simulink model "TBRe19_ECU_Torque_request_TSS_ON"  (R2017b)
settings: Solver=FixedStepDiscrete  StartTime=0.0  StopTime=inf  FixedStep=0.0001  RelTol=1e-3
PostLoadFcn:
  | model_init();
libraries: simulink x17
(part 2 of 6)

== system TBRe19_ECU_Torque_request_TSS_ON/MainTask/Comms_And_Data_Acquisition_Layer/MCU_CAN ==
  note: Overall Functionality:
      | Read CAN messages related to motor control unit (MCU)
  Bus Creator1 : BusCreator  Inputs=4
  CanRx1 : S-Function  FunctionName=NsiCan_Rx_J1939_Ext  Parameters=data_can,channel,msg_name,ident,ident_type,dlc,signals,is_trigger,is_SA_Masked,is_TA_Masked,is_physical,is_canfd  SFunctionDeploymentMode=off  EnableBusSupport=off  mask(MUXlink Can Rx){data_can=1;HIGH_SPEED;500Kbps;No;C:\Users\TBRe-admin\Documents\TBReVCU\TBRe19_DBC.dbc;0;;;0;HIGH_SPEED;500Kbps;120 Ohm;C:\Users\TBRe-admin\Documents\Database\TBRe19_DBC_190517.dbc;0;;;0;HIGH_SPEED;1000Kbps;120 Ohm;D:\TOOLS\MUXLINK\R2011b\MUXlink\misc\BASE_CAN_MUXLAB4.dbc;0;;;0;HIGH_SPEED;500Kbps;120 Ohm;D:\TOOLS\MUXLINK\R2011b\MUXlink\misc\j1939_adapt.dbc;0;;;0;HIGH_SPEED;1000Kbps;No;D:\TOOLS\MUXLINK\R2011b\MUXlink\misc\BASE_CAN_MUXLAB4.dbc;0;;, channel=1, msg_name=HS3_Temperature_Feedback, ident=0x191AFF71, ident_type=XTD, dlc=8, signals=DC_Link_Voltage;1;32;-16;0.062500;0.000000;V;MotorTemperature;1;16;-16;1.000000;0.000000;C, is_trigger=0, is_physical=1, is_canfd=0, is_SA_Masked=1, is_TA_Masked=0}
      mask prompts: data_can "data can"; msg_name "msg name"; is_SA_Masked "J1939 SA filtering"; is_TA_Masked "J1939 TA filtering"
      mask help: Receive a frame from a CAN channel.
      mask init:
      | NsiCan_Rx_J1939_Ext_InitializationFcn();
      settings: OpenFcn=NsiCan_Rx_J1939_Ext_OpenFcn();
      mask Help:
      | eval('block=get_param(gcb, ''RTWdata'');')
      | web([docroot '\toolbox\MUXlink\html\blocks/' block.MUXlink_BlockType '.html'])
      mask Callback data_can: NsiCan_Rx_J1939_Ext_ApplyFcn(1);
      mask Callback channel: NsiCan_Rx_J1939_Ext_ApplyFcn(2);
      mask Callback msg_name: NsiCan_Rx_J1939_Ext_ApplyFcn(3);
      mask Callback ident: NsiCan_Rx_J1939_Ext_ApplyFcn(4);
      mask Callback ident_type: NsiCan_Rx_J1939_Ext_ApplyFcn(5);
      mask Callback dlc: NsiCan_Rx_J1939_Ext_ApplyFcn(6);
      mask Callback signals: NsiCan_Rx_J1939_Ext_ApplyFcn(7);
      mask Callback is_trigger: NsiCan_Rx_J1939_Ext_ApplyFcn(8);
      mask Callback is_physical: NsiCan_Rx_J1939_Ext_ApplyFcn(9);
      mask Callback is_canfd: NsiCan_Rx_J1939_Ext_ApplyFcn(10);
      mask Callback is_SA_Masked: NsiCan_Rx_J1939_Ext_ApplyFcn(11);
      mask Callback is_TA_Masked: NsiCan_Rx_J1939_Ext_ApplyFcn(12);
      mask Display: image(imread('nsi.bmp'));text(0.5, 0.3, 'J1939_PGN  HS3_Temperature_Feedbackchannel CAN1', 'horizontalAlignment', 'center', 'verticalAlignment', 'base');plot([0.05 0.05 0.05 0.05 0.05 0.05 0.05 0.05 0.05 0.05]); port_label('output',1, 'DC_Link_Voltage'); port_label('output',2, 'MotorTemperature'); port_label('output',3, 'Status');
  CanRx2 : S-Function  FunctionName=NsiCan_Rx_J1939_Ext  Parameters=data_can,channel,msg_name,ident,ident_type,dlc,signals,is_trigger,is_SA_Masked,is_TA_Masked,is_physical,is_canfd  SFunctionDeploymentMode=off  EnableBusSupport=off  mask(MUXlink Can Rx){data_can=1;HIGH_SPEED;500Kbps;No;C:\Users\TBRe-admin\Documents\TBReVCU\TBRe19_DBC.dbc;0;;;0;HIGH_SPEED;500Kbps;120 Ohm;C:\Users\TBRe-admin\Documents\Database\TBRe19_DBC_190517.dbc;0;;;0;HIGH_SPEED;1000Kbps;120 Ohm;D:\TOOLS\MUXLINK\R2011b\MUXlink\misc\BASE_CAN_MUXLAB4.dbc;0;;;0;HIGH_SPEED;500Kbps;120 Ohm;D:\TOOLS\MUXLINK\R2011b\MUXlink\misc\j1939_adapt.dbc;0;;;0;HIGH_SPEED;1000Kbps;No;D:\TOOLS\MUXLINK\R2011b\MUXlink\misc\BASE_CAN_MUXLAB4.dbc;0;;, channel=1, msg_name=HD4_Debug_Temperatures_B, ident=0x192BFF71, ident_type=XTD, dlc=8, signals=Debug_Temps_Heatsink;1;24;8;1.000000;0.000000;degC, is_trigger=0, is_physical=1, is_canfd=0, is_SA_Masked=1, is_TA_Masked=0}
      mask prompts: data_can "data can"; msg_name "msg name"; is_SA_Masked "J1939 SA filtering"; is_TA_Masked "J1939 TA filtering"
      mask help: Receive a frame from a CAN channel.
      mask init:
      | NsiCan_Rx_J1939_Ext_InitializationFcn();
      settings: OpenFcn=NsiCan_Rx_J1939_Ext_OpenFcn();
      mask Help:
      | eval('block=get_param(gcb, ''RTWdata'');')
      | web([docroot '\toolbox\MUXlink\html\blocks/' block.MUXlink_BlockType '.html'])
      mask Callback data_can: NsiCan_Rx_J1939_Ext_ApplyFcn(1);
      mask Callback channel: NsiCan_Rx_J1939_Ext_ApplyFcn(2);
      mask Callback msg_name: NsiCan_Rx_J1939_Ext_ApplyFcn(3);
      mask Callback ident: NsiCan_Rx_J1939_Ext_ApplyFcn(4);
      mask Callback ident_type: NsiCan_Rx_J1939_Ext_ApplyFcn(5);
      mask Callback dlc: NsiCan_Rx_J1939_Ext_ApplyFcn(6);
      mask Callback signals: NsiCan_Rx_J1939_Ext_ApplyFcn(7);
      mask Callback is_trigger: NsiCan_Rx_J1939_Ext_ApplyFcn(8);
      mask Callback is_physical: NsiCan_Rx_J1939_Ext_ApplyFcn(9);
      mask Callback is_canfd: NsiCan_Rx_J1939_Ext_ApplyFcn(10);
      mask Callback is_SA_Masked: NsiCan_Rx_J1939_Ext_ApplyFcn(11);
      mask Callback is_TA_Masked: NsiCan_Rx_J1939_Ext_ApplyFcn(12);
      mask Display: image(imread('nsi.bmp'));text(0.5, 0.3, 'J1939_PGN  HD4_Debug_Temperatures_Bchannel CAN1', 'horizontalAlignment', 'center', 'verticalAlignment', 'base');plot([0.05 0.05 0.05 0.05 0.05 0.05 0.05 0.05 0.05 0.05]); port_label('output',1, 'Debug_Temps_Heatsink'); port_label('output',2, 'Status');
  CanRx3 : S-Function  FunctionName=NsiCan_Rx_J1939_Ext  Parameters=data_can,channel,msg_name,ident,ident_type,dlc,signals,is_trigger,is_SA_Masked,is_TA_Masked,is_physical,is_canfd  SFunctionDeploymentMode=off  EnableBusSupport=off  mask(MUXlink Can Rx){data_can=1;HIGH_SPEED;500Kbps;No;C:\Users\TBRe-admin\Documents\TBReVCU\TBRe19_DBC.dbc;0;;;0;HIGH_SPEED;500Kbps;120 Ohm;C:\Users\TBRe-admin\Documents\Database\TBRe19_DBC_190517.dbc;0;;;0;HIGH_SPEED;1000Kbps;120 Ohm;D:\TOOLS\MUXLINK\R2011b\MUXlink\misc\BASE_CAN_MUXLAB4.dbc;0;;;0;HIGH_SPEED;500Kbps;120 Ohm;D:\TOOLS\MUXLINK\R2011b\MUXlink\misc\j1939_adapt.dbc;0;;;0;HIGH_SPEED;1000Kbps;No;D:\TOOLS\MUXLINK\R2011b\MUXlink\misc\BASE_CAN_MUXLAB4.dbc;0;;, channel=1, msg_name=HS1_Torque_Feedback, ident=0x1918FF71, ident_type=XTD, dlc=8, signals=Speed_Measured;1;16;-16;1.000000;0.000000;RPM;Torque_Measured;1;0;-16;0.062500;0.000000;Nm, is_trigger=0, is_physical=1, is_canfd=0, is_SA_Masked=1, is_TA_Masked=0}
      mask prompts: data_can "data can"; msg_name "msg name"; is_SA_Masked "J1939 SA filtering"; is_TA_Masked "J1939 TA filtering"
      mask help: Receive a frame from a CAN channel.
      mask init:
      | NsiCan_Rx_J1939_Ext_InitializationFcn();
      settings: OpenFcn=NsiCan_Rx_J1939_Ext_OpenFcn();
      mask Help:
      | eval('block=get_param(gcb, ''RTWdata'');')
      | web([docroot '\toolbox\MUXlink\html\blocks/' block.MUXlink_BlockType '.html'])
      mask Callback data_can: NsiCan_Rx_J1939_Ext_ApplyFcn(1);
      mask Callback channel: NsiCan_Rx_J1939_Ext_ApplyFcn(2);
      mask Callback msg_name: NsiCan_Rx_J1939_Ext_ApplyFcn(3);
      mask Callback ident: NsiCan_Rx_J1939_Ext_ApplyFcn(4);
      mask Callback ident_type: NsiCan_Rx_J1939_Ext_ApplyFcn(5);
      mask Callback dlc: NsiCan_Rx_J1939_Ext_ApplyFcn(6);
      mask Callback signals: NsiCan_Rx_J1939_Ext_ApplyFcn(7);
      mask Callback is_trigger: NsiCan_Rx_J1939_Ext_ApplyFcn(8);
      mask Callback is_physical: NsiCan_Rx_J1939_Ext_ApplyFcn(9);
      mask Callback is_canfd: NsiCan_Rx_J1939_Ext_ApplyFcn(10);
      mask Callback is_SA_Masked: NsiCan_Rx_J1939_Ext_ApplyFcn(11);
      mask Callback is_TA_Masked: NsiCan_Rx_J1939_Ext_ApplyFcn(12);
      mask Display: image(imread('nsi.bmp'));text(0.5, 0.3, 'J1939_PGN  HS1_Torque_Feedbackchannel CAN1', 'horizontalAlignment', 'center', 'verticalAlignment', 'base');plot([0.05 0.05 0.05 0.05 0.05 0.05 0.05 0.05 0.05 0.05]); port_label('output',1, 'Speed_Measured'); port_label('output',2, 'Torque_Measured'); port_label('output',3, 'Status');
  Data Type Conversion : DataTypeConversion  OutDataTypeStr=int16
  Terminator : Terminator
  Terminator1 : Terminator
  Terminator2 : Terminator
  UsbTx1 : S-Function  FunctionName=NsiUsb_Tx  Parameters=signame,resolution,offset,unite  SFunctionDeploymentMode=off  EnableBusSupport=off  mask(MUXlink Usb Tx){signame=MCU_V, resolution=1, offset=0, unite=V}
      mask prompts: signame "Signal name ?"; resolution "Resolution ?"; offset "Offset ?"; unite "Unit ?"
      mask help: Transmit a frame on the USB Channel.
      mask init:
      | NsiUsb_Tx_InitializationFcn();
      settings: OpenFcn=NsiUsb_Tx_OpenFcn();
      mask Help:
      | eval('block=get_param(gcb, ''RTWdata'');')
      | web([docroot '\toolbox\MUXlink\html\blocks/' block.MUXlink_BlockType '.html'])
      mask Callback signame: NsiUsb_Tx_ApplyFcn(1);
      mask Callback resolution: NsiUsb_Tx_ApplyFcn(2);
      mask Callback offset: NsiUsb_Tx_ApplyFcn(3);
      mask Callback unite: NsiUsb_Tx_ApplyFcn(4);
      mask Display: image(imread('nsi.bmp'));text(0.5, 0.2, 'USB Tx', 'horizontalAlignment', 'center', 'verticalAlignment', 'base');plot([0.05 0.05 0.05 0.05 0.05 0.05 0.05 0.05 0.05 0.05]);port_label('input',1, 'MCU_V');
  UsbTx2 : S-Function  FunctionName=NsiUsb_Tx  Parameters=signame,resolution,offset,unite  SFunctionDeploymentMode=off  EnableBusSupport=off  mask(MUXlink Usb Tx){signame=Motor_Temp, resolution=1, offset=0, unite=Degrees}
      mask prompts: signame "Signal name ?"; resolution "Resolution ?"; offset "Offset ?"; unite "Unit ?"
      mask help: Transmit a frame on the USB Channel.
      mask init:
      | NsiUsb_Tx_InitializationFcn();
      settings: OpenFcn=NsiUsb_Tx_OpenFcn();
      mask Help:
      | eval('block=get_param(gcb, ''RTWdata'');')
      | web([docroot '\toolbox\MUXlink\html\blocks/' block.MUXlink_BlockType '.html'])
      mask Callback signame: NsiUsb_Tx_ApplyFcn(1);
      mask Callback resolution: NsiUsb_Tx_ApplyFcn(2);
      mask Callback offset: NsiUsb_Tx_ApplyFcn(3);
      mask Callback unite: NsiUsb_Tx_ApplyFcn(4);
      mask Display: image(imread('nsi.bmp'));text(0.5, 0.2, 'USB Tx', 'horizontalAlignment', 'center', 'verticalAlignment', 'base');plot([0.05 0.05 0.05 0.05 0.05 0.05 0.05 0.05 0.05 0.05]);port_label('input',1, 'Motor_Temp');
  UsbTx3 : S-Function  FunctionName=NsiUsb_Tx  Parameters=signame,resolution,offset,unite  SFunctionDeploymentMode=off  EnableBusSupport=off  mask(MUXlink Usb Tx){signame=MCU_Temp, resolution=1, offset=0, unite=Degrees}
      mask prompts: signame "Signal name ?"; resolution "Resolution ?"; offset "Offset ?"; unite "Unit ?"
      mask help: Transmit a frame on the USB Channel.
      mask init:
      | NsiUsb_Tx_InitializationFcn();
      settings: OpenFcn=NsiUsb_Tx_OpenFcn();
      mask Help:
      | eval('block=get_param(gcb, ''RTWdata'');')
      | web([docroot '\toolbox\MUXlink\html\blocks/' block.MUXlink_BlockType '.html'])
      mask Callback signame: NsiUsb_Tx_ApplyFcn(1);
      mask Callback resolution: NsiUsb_Tx_ApplyFcn(2);
      mask Callback offset: NsiUsb_Tx_ApplyFcn(3);
      mask Callback unite: NsiUsb_Tx_ApplyFcn(4);
      mask Display: image(imread('nsi.bmp'));text(0.5, 0.2, 'USB Tx', 'horizontalAlignment', 'center', 'verticalAlignment', 'base');plot([0.05 0.05 0.05 0.05 0.05 0.05 0.05 0.05 0.05 0.05]);port_label('input',1, 'MCU_Temp');
  UsbTx4 : S-Function  FunctionName=NsiUsb_Tx  Parameters=signame,resolution,offset,unite  SFunctionDeploymentMode=off  EnableBusSupport=off  mask(MUXlink Usb Tx){signame=MotorSpeed, resolution=1, offset=0, unite=RPM}
      mask prompts: signame "Signal name ?"; resolution "Resolution ?"; offset "Offset ?"; unite "Unit ?"
      mask help: Transmit a frame on the USB Channel.
      mask init:
      | NsiUsb_Tx_InitializationFcn();
      settings: OpenFcn=NsiUsb_Tx_OpenFcn();
      mask Help:
      | eval('block=get_param(gcb, ''RTWdata'');')
      | web([docroot '\toolbox\MUXlink\html\blocks/' block.MUXlink_BlockType '.html'])
      mask Callback signame: NsiUsb_Tx_ApplyFcn(1);
      mask Callback resolution: NsiUsb_Tx_ApplyFcn(2);
      mask Callback offset: NsiUsb_Tx_ApplyFcn(3);
      mask Callback unite: NsiUsb_Tx_ApplyFcn(4);
      mask Display: image(imread('nsi.bmp'));text(0.5, 0.2, 'USB Tx', 'horizontalAlignment', 'center', 'verticalAlignment', 'base');plot([0.05 0.05 0.05 0.05 0.05 0.05 0.05 0.05 0.05 0.05]);port_label('input',1, 'MotorSpeed');
  HAL_MCU : Outport
  wires:
  Bus Creator1/1 -> HAL_MCU/1  "HAL_MCU"
  CanRx1/1 -> UsbTx1/1, Bus Creator1/1  "MCU_Voltage"
  CanRx1/2 -> UsbTx2/1, Bus Creator1/2  "Motor_Temp"
  CanRx2/1 -> UsbTx3/1, Bus Creator1/3  "MCU_Temp"
  CanRx3/1 -> Data Type Conversion/1  "Motor_Speed"
  CanRx1/3 -> Terminator/1  "MCU_Temp"
  CanRx2/2 -> Terminator1/1
  CanRx3/2 -> Terminator2/1
  Data Type Conversion/1 -> UsbTx4/1, Bus Creator1/4  "Motor_Speed"

== system TBRe19_ECU_Torque_request_TSS_ON/MainTask/Comms_And_Data_Acquisition_Layer/SENSOR_CAN ==
  note: Overall Functionality:
      | Read CAN messages related to vehicle sensors
  Bus Creator3 : BusCreator  Inputs=9
  CanRx5 : S-Function  FunctionName=NsiCan_Rx_Ext  Parameters=data_can,channel,msg_name,ident,ident_type,dlc,signals,is_trigger,is_physical,is_canfd,is_rxgw  SFunctionDeploymentMode=off  EnableBusSupport=off  mask(MUXlink Can Rx){data_can=1;HIGH_SPEED;500Kbps;No;C:\Users\TBRe-admin\Documents\TBReVCU\TBRe19_DBC.dbc;0;;;0;HIGH_SPEED;500Kbps;120 Ohm;C:\Users\TBRe-admin\Documents\Database\TBRe19_DBC_190517.dbc;0;;;0;HIGH_SPEED;1000Kbps;120 Ohm;D:\TOOLS\MUXLINK\R2011b\MUXlink\misc\BASE_CAN_MUXLAB4.dbc;0;;;0;HIGH_SPEED;500Kbps;120 Ohm;D:\TOOLS\MUXLINK\R2011b\MUXlink\misc\j1939_adapt.dbc;0;;;0;HIGH_SPEED;1000Kbps;No;D:\TOOLS\MUXLINK\R2011b\MUXlink\misc\BASE_CAN_MUXLAB4.dbc;0;;, channel=1, msg_name=SteeringWheelSensor, ident=0x234, ident_type=STD, dlc=5, signals=Acc_Angle;1;0;-16;0.100000;0.000000;Degrees, is_trigger=0, is_physical=1, is_canfd=0, is_rxgw=0}
      mask prompts: data_can "data can"; msg_name "msg name"
      mask help: Receive a frame from a CAN channel.
      mask init:
      | NsiCan_Rx_Ext_InitializationFcn();
      settings: OpenFcn=NsiCan_Rx_Ext_OpenFcn();
      mask Help:
      | eval('block=get_param(gcb, ''RTWdata'');')
      | web([docroot '\toolbox\MUXlink\html\blocks/' block.MUXlink_BlockType '.html'])
      mask Callback data_can: NsiCan_Rx_Ext_ApplyFcn(1);
      mask Callback channel: NsiCan_Rx_Ext_ApplyFcn(2);
      mask Callback msg_name: NsiCan_Rx_Ext_ApplyFcn(3);
      mask Callback ident: NsiCan_Rx_Ext_ApplyFcn(4);
      mask Callback ident_type: NsiCan_Rx_Ext_ApplyFcn(5);
      mask Callback dlc: NsiCan_Rx_Ext_ApplyFcn(6);
      mask Callback signals: NsiCan_Rx_Ext_ApplyFcn(7);
      mask Callback is_trigger: NsiCan_Rx_Ext_ApplyFcn(8);
      mask Callback is_physical: NsiCan_Rx_Ext_ApplyFcn(9);
      mask Callback is_canfd: NsiCan_Rx_Ext_ApplyFcn(10);
      mask Callback is_rxgw: NsiCan_Rx_Ext_ApplyFcn(11);
      mask Display: image(imread('nsi.bmp'));text(0.5, 0.3, 'RX_SteeringWheelSensor_CAN1', 'horizontalAlignment', 'center', 'verticalAlignment', 'base');plot([0.05 0.05 0.05 0.05 0.05 0.05 0.05 0.05 0.05 0.05]); port_label('output',1, 'Acc_Angle'); port_label('output',2, 'Status');
  CanRx8 : S-Function  FunctionName=NsiCan_Rx_Ext  Parameters=data_can,channel,msg_name,ident,ident_type,dlc,signals,is_trigger,is_physical,is_canfd,is_rxgw  SFunctionDeploymentMode=off  EnableBusSupport=off  mask(MUXlink Can Rx){data_can=1;HIGH_SPEED;500Kbps;No;C:\Users\TBRe-admin\Documents\TBReVCU\TBRe19_DBC.dbc;0;;;0;HIGH_SPEED;500Kbps;120 Ohm;C:\Users\TBRe-admin\Documents\Database\TBRe19_DBC_190517.dbc;0;;;0;HIGH_SPEED;1000Kbps;120 Ohm;D:\TOOLS\MUXLINK\R2011b\MUXlink\misc\BASE_CAN_MUXLAB4.dbc;0;;;0;HIGH_SPEED;500Kbps;120 Ohm;D:\TOOLS\MUXLINK\R2011b\MUXlink\misc\j1939_adapt.dbc;0;;;0;HIGH_SPEED;1000Kbps;No;D:\TOOLS\MUXLINK\R2011b\MUXlink\misc\BASE_CAN_MUXLAB4.dbc;0;;, channel=1, msg_name=AccelerometerY, ident=0x174, ident_type=STD, dlc=8, signals=Acc_Yaw;1;0;16;0.005000;0.000000;_, is_trigger=0, is_physical=1, is_canfd=0, is_rxgw=0}
      mask prompts: data_can "data can"; msg_name "msg name"
      mask help: Receive a frame from a CAN channel.
      mask init:
      | NsiCan_Rx_Ext_InitializationFcn();
      settings: OpenFcn=NsiCan_Rx_Ext_OpenFcn();
      mask Help:
      | eval('block=get_param(gcb, ''RTWdata'');')
      | web([docroot '\toolbox\MUXlink\html\blocks/' block.MUXlink_BlockType '.html'])
      mask Callback data_can: NsiCan_Rx_Ext_ApplyFcn(1);
      mask Callback channel: NsiCan_Rx_Ext_ApplyFcn(2);
      mask Callback msg_name: NsiCan_Rx_Ext_ApplyFcn(3);
      mask Callback ident: NsiCan_Rx_Ext_ApplyFcn(4);
      mask Callback ident_type: NsiCan_Rx_Ext_ApplyFcn(5);
      mask Callback dlc: NsiCan_Rx_Ext_ApplyFcn(6);
      mask Callback signals: NsiCan_Rx_Ext_ApplyFcn(7);
      mask Callback is_trigger: NsiCan_Rx_Ext_ApplyFcn(8);
      mask Callback is_physical: NsiCan_Rx_Ext_ApplyFcn(9);
      mask Callback is_canfd: NsiCan_Rx_Ext_ApplyFcn(10);
      mask Callback is_rxgw: NsiCan_Rx_Ext_ApplyFcn(11);
      mask Display: image(imread('nsi.bmp'));text(0.5, 0.3, 'RX_AccelerometerY_CAN1', 'horizontalAlignment', 'center', 'verticalAlignment', 'base');plot([0.05 0.05 0.05 0.05 0.05 0.05 0.05 0.05 0.05 0.05]); port_label('output',1, 'Acc_Yaw'); port_label('output',2, 'Status');
  CanRx9 : S-Function  FunctionName=NsiCan_Rx_Ext  Parameters=data_can,channel,msg_name,ident,ident_type,dlc,signals,is_trigger,is_physical,is_canfd,is_rxgw  SFunctionDeploymentMode=off  EnableBusSupport=off  mask(MUXlink Can Rx){data_can=1;HIGH_SPEED;500Kbps;No;C:\Users\TBRe-admin\Documents\TBReVCU\TBRe19_DBC.dbc;0;;;0;HIGH_SPEED;500Kbps;120 Ohm;C:\Users\TBRe-admin\Documents\Database\TBRe19_DBC_190517.dbc;0;;;0;HIGH_SPEED;1000Kbps;120 Ohm;D:\TOOLS\MUXLINK\R2011b\MUXlink\misc\BASE_CAN_MUXLAB4.dbc;0;;;0;HIGH_SPEED;500Kbps;120 Ohm;D:\TOOLS\MUXLINK\R2011b\MUXlink\misc\j1939_adapt.dbc;0;;;0;HIGH_SPEED;1000Kbps;No;D:\TOOLS\MUXLINK\R2011b\MUXlink\misc\BASE_CAN_MUXLAB4.dbc;0;;, channel=1, msg_name=Shutdown_Data, ident=0x705, ident_type=STD, dlc=3, signals=Fault_CarShutdown;1;0;1;1.000000;0.000000;_, is_trigger=0, is_physical=1, is_canfd=0, is_rxgw=0}
      mask prompts: data_can "data can"; msg_name "msg name"
      mask help: Receive a frame from a CAN channel.
      mask init:
      | NsiCan_Rx_Ext_InitializationFcn();
      settings: OpenFcn=NsiCan_Rx_Ext_OpenFcn();
      mask Help:
      | eval('block=get_param(gcb, ''RTWdata'');')
      | web([docroot '\toolbox\MUXlink\html\blocks/' block.MUXlink_BlockType '.html'])
      mask Callback data_can: NsiCan_Rx_Ext_ApplyFcn(1);
      mask Callback channel: NsiCan_Rx_Ext_ApplyFcn(2);
      mask Callback msg_name: NsiCan_Rx_Ext_ApplyFcn(3);
      mask Callback ident: NsiCan_Rx_Ext_ApplyFcn(4);
      mask Callback ident_type: NsiCan_Rx_Ext_ApplyFcn(5);
      mask Callback dlc: NsiCan_Rx_Ext_ApplyFcn(6);
      mask Callback signals: NsiCan_Rx_Ext_ApplyFcn(7);
      mask Callback is_trigger: NsiCan_Rx_Ext_ApplyFcn(8);
      mask Callback is_physical: NsiCan_Rx_Ext_ApplyFcn(9);
      mask Callback is_canfd: NsiCan_Rx_Ext_ApplyFcn(10);
      mask Callback is_rxgw: NsiCan_Rx_Ext_ApplyFcn(11);
      mask Display: image(imread('nsi.bmp'));text(0.5, 0.3, 'RX_Shutdown_Data_CAN1', 'horizontalAlignment', 'center', 'verticalAlignment', 'base');plot([0.05 0.05 0.05 0.05 0.05 0.05 0.05 0.05 0.05 0.05]); port_label('output',1, 'Fault_CarShutdown'); port_label('output',2, 'Status');
  Terminator2 : Terminator
  Terminator3 : Terminator
  Terminator4 : Terminator
  Sensor_Data : Outport
  wires:
  CanRx5/2 -> Terminator2/1
  CanRx8/2 -> Terminator3/1
  CanRx9/2 -> Terminator4/1
  CanRx9/1 -> Bus Creator3/9  "Shutdown_Error"
  CanRx5/1 -> Bus Creator3/7  "Steering_Angle"
  CanRx8/1 -> Bus Creator3/8  "Yaw"
  Bus Creator3/1 -> Sensor_Data/1  "Sensor_Data"

== system TBRe19_ECU_Torque_request_TSS_ON/MainTask/Comms_And_Data_Output_Layer/Hardwired_Ouputs ==
  note: ECU Ok Ouput
  note: TSS Output
  note: Turns the MCU on
  note: Accy Fan
  note: Pump and Fan
  PostPL_Data : Inport
  AnalogOutput1 : S-Function  Description=This block interface the 8 Analog Outputs. The analog outputs are 0/20V. Voltage input is set in mV  FunctionName=NsiIo_AnalogOutput  Parameters=Channel,Feedback  SFunctionDeploymentMode=off  EnableBusSupport=off  mask(MUXlink I/O Analog Output){Channel=2, Feedback=off, RANGE=0 / 20 Volts}
      mask prompts: Channel "Channel ?"; Feedback "Read Back Analog out"; RANGE "Voltage Range"
      mask help: This block interface the 8 Analog Outputs. Channels 1 to 4 are 0/10V, and the channels 5 to 8 are0/20V. Voltage input is set in mV
      mask init:
      | NsiIo_AnalogOutput_InitializationFcn();
      settings: OpenFcn=NsiIo_AnalogOutput_OpenFcn();
      mask Help:
      | eval('block=get_param(gcb, ''RTWdata'');')
      | web([docroot '\toolbox\MUXlink\html\blocks/' block.MUXlink_BlockType '.html'])
      mask Callback Channel: NsiIo_AnalogOutput_ApplyFcn(1);
      mask Display: image(imread('nsi.bmp'));text(0.5, 0.2, 'AnalogOutput_2\n\n0 / 20 Volts', 'horizontalAlignment', 'center', 'verticalAlignment', 'base');plot([0.05 0.05 0.05 0.05 0.05 0.05 0.05 0.05 0.05 0.05]);port_label('input', 1, 'E4');
  AnalogOutput2 : S-Function  Description=This block interface the 8 Analog Outputs. The analog outputs are 0/20V. Voltage input is set in mV  FunctionName=NsiIo_AnalogOutput  Parameters=Channel,Feedback  SFunctionDeploymentMode=off  EnableBusSupport=off  mask(MUXlink I/O Analog Output){Channel=1, Feedback=off, RANGE=0 / 20 Volts}
      mask prompts: Channel "Channel ?"; Feedback "Read Back Analog out"; RANGE "Voltage Range"
      mask help: This block interface the 8 Analog Outputs. Channels 1 to 4 are 0/10V, and the channels 5 to 8 are0/20V. Voltage input is set in mV
      mask init:
      | NsiIo_AnalogOutput_InitializationFcn();
      settings: OpenFcn=NsiIo_AnalogOutput_OpenFcn();
      mask Help:
      | eval('block=get_param(gcb, ''RTWdata'');')
      | web([docroot '\toolbox\MUXlink\html\blocks/' block.MUXlink_BlockType '.html'])
      mask Callback Channel: NsiIo_AnalogOutput_ApplyFcn(1);
      mask Display: image(imread('nsi.bmp'));text(0.5, 0.2, 'AnalogOutput_1\n\n0 / 20 Volts', 'horizontalAlignment', 'center', 'verticalAlignment', 'base');plot([0.05 0.05 0.05 0.05 0.05 0.05 0.05 0.05 0.05 0.05]);port_label('input', 1, 'E3');
  Bus Selector : BusSelector  OutputSignals=Hardwired_Peripherals.Coolant_Enable,Hardwired_Peripherals.PumpFanPower,Hardwired_Peripherals.AccyFanPower,Hardwired_Peripherals.Brake_Light,Hardwired_Peripherals.Buzzer,Hardwired_Peripherals.ECU_Ok,Hardwired_Peripherals.TSS
  DigitalOutput2 : S-Function  FunctionName=NsiIo_DigitalOutput  Parameters=channel,side,feedback  SFunctionDeploymentMode=off  EnableBusSupport=off  mask(MUXlink I/O Digital Output){channel=1, side=High, feedback=off}
      mask prompts: channel "Channel ?"; side "Side ?"; feedback "With feedback ?"
      mask help: Write Digital Output onto I/O channel.
      mask init:
      | NsiIo_DigitalOutput_InitializationFcn();
      settings: OpenFcn=NsiIo_DigitalOutput_OpenFcn();
      mask Help:
      | eval('block=get_param(gcb, ''RTWdata'');')
      | web([docroot '\toolbox\MUXlink\html\blocks/' block.MUXlink_BlockType '.html'])
      mask Callback channel: NsiIo_DigitalOutput_ApplyFcn(1);
      mask TypeOptions side: High | Low
      mask Callback side: NsiIo_DigitalOutput_ApplyFcn(2);
      mask Callback feedback: NsiIo_DigitalOutput_ApplyFcn(3);
      mask Display: image(imread('nsi.bmp'));text(0.5, 0.2, 'DigitalOutput_1', 'horizontalAlignment', 'center', 'verticalAlignment', 'base');plot([0.05 0.05 0.05 0.05 0.05 0.05 0.05 0.05 0.05 0.05]);port_label('input', 1, 'G2 : High Side');
  DigitalOutput3 : S-Function  FunctionName=NsiIo_DigitalOutput  Parameters=channel,side,feedback  SFunctionDeploymentMode=off  EnableBusSupport=off  mask(MUXlink I/O Digital Output){channel=7, side=Low, feedback=off}
      mask prompts: channel "Channel ?"; side "Side ?"; feedback "With feedback ?"
      mask help: Write Digital Output onto I/O channel.
      mask init:
      | NsiIo_DigitalOutput_InitializationFcn();
      settings: OpenFcn=NsiIo_DigitalOutput_OpenFcn();
      mask Help:
      | eval('block=get_param(gcb, ''RTWdata'');')
      | web([docroot '\toolbox\MUXlink\html\blocks/' block.MUXlink_BlockType '.html'])
      mask Callback channel: NsiIo_DigitalOutput_ApplyFcn(1);
      mask TypeOptions side: High | Low
      mask Callback side: NsiIo_DigitalOutput_ApplyFcn(2);
      mask Callback feedback: NsiIo_DigitalOutput_ApplyFcn(3);
      mask Display: image(imread('nsi.bmp'));text(0.5, 0.2, 'DigitalOutput_7', 'horizontalAlignment', 'center', 'verticalAlignment', 'base');plot([0.05 0.05 0.05 0.05 0.05 0.05 0.05 0.05 0.05 0.05]);port_label('input', 1, 'H2 : Low Side');
  DigitalOutput4 : S-Function  FunctionName=NsiIo_DigitalOutput  Parameters=channel,side,feedback  SFunctionDeploymentMode=off  EnableBusSupport=off  mask(MUXlink I/O Digital Output){channel=4, side=High, feedback=off}
      mask prompts: channel "Channel ?"; side "Side ?"; feedback "With feedback ?"
      mask help: Write Digital Output onto I/O channel.
      mask init:
      | NsiIo_DigitalOutput_InitializationFcn();
      settings: OpenFcn=NsiIo_DigitalOutput_OpenFcn();
      mask Help:
      | eval('block=get_param(gcb, ''RTWdata'');')
      | web([docroot '\toolbox\MUXlink\html\blocks/' block.MUXlink_BlockType '.html'])
      mask Callback channel: NsiIo_DigitalOutput_ApplyFcn(1);
      mask TypeOptions side: High | Low
      mask Callback side: NsiIo_DigitalOutput_ApplyFcn(2);
      mask Callback feedback: NsiIo_DigitalOutput_ApplyFcn(3);
      mask Display: image(imread('nsi.bmp'));text(0.5, 0.2, 'DigitalOutput_4', 'horizontalAlignment', 'center', 'verticalAlignment', 'base');plot([0.05 0.05 0.05 0.05 0.05 0.05 0.05 0.05 0.05 0.05]);port_label('input', 1, 'L4 : High Side');
  DigitalOutput5 : S-Function  FunctionName=NsiIo_DigitalOutput  Parameters=channel,side,feedback  SFunctionDeploymentMode=off  EnableBusSupport=off  mask(MUXlink I/O Digital Output){channel=6, side=High, feedback=off}
      mask prompts: channel "Channel ?"; side "Side ?"; feedback "With feedback ?"
      mask help: Write Digital Output onto I/O channel.
      mask init:
      | NsiIo_DigitalOutput_InitializationFcn();
      settings: OpenFcn=NsiIo_DigitalOutput_OpenFcn();
      mask Help:
      | eval('block=get_param(gcb, ''RTWdata'');')
      | web([docroot '\toolbox\MUXlink\html\blocks/' block.MUXlink_BlockType '.html'])
      mask Callback channel: NsiIo_DigitalOutput_ApplyFcn(1);
      mask TypeOptions side: High | Low
      mask Callback side: NsiIo_DigitalOutput_ApplyFcn(2);
      mask Callback feedback: NsiIo_DigitalOutput_ApplyFcn(3);
      mask Display: image(imread('nsi.bmp'));text(0.5, 0.2, 'DigitalOutput_6', 'horizontalAlignment', 'center', 'verticalAlignment', 'base');plot([0.05 0.05 0.05 0.05 0.05 0.05 0.05 0.05 0.05 0.05]);port_label('input', 1, 'M4 : High Side');
  DigitalOutput6 : S-Function  FunctionName=NsiIo_DigitalOutput  Parameters=channel,side,feedback  SFunctionDeploymentMode=off  EnableBusSupport=off  mask(MUXlink I/O Digital Output){channel=3, side=High, feedback=off}
      mask prompts: channel "Channel ?"; side "Side ?"; feedback "With feedback ?"
      mask help: Write Digital Output onto I/O channel.
      mask init:
      | NsiIo_DigitalOutput_InitializationFcn();
      settings: OpenFcn=NsiIo_DigitalOutput_OpenFcn();
      mask Help:
      | eval('block=get_param(gcb, ''RTWdata'');')
      | web([docroot '\toolbox\MUXlink\html\blocks/' block.MUXlink_BlockType '.html'])
      mask Callback channel: NsiIo_DigitalOutput_ApplyFcn(1);
      mask TypeOptions side: High | Low
      mask Callback side: NsiIo_DigitalOutput_ApplyFcn(2);
      mask Callback feedback: NsiIo_DigitalOutput_ApplyFcn(3);
      mask Display: image(imread('nsi.bmp'));text(0.5, 0.2, 'DigitalOutput_3', 'horizontalAlignment', 'center', 'verticalAlignment', 'base');plot([0.05 0.05 0.05 0.05 0.05 0.05 0.05 0.05 0.05 0.05]);port_label('input', 1, 'L3 : High Side');
  DigitalOutput7 : S-Function  FunctionName=NsiIo_DigitalOutput  Parameters=channel,side,feedback  SFunctionDeploymentMode=off  EnableBusSupport=off  mask(MUXlink I/O Digital Output){channel=5, side=High, feedback=off}
      mask prompts: channel "Channel ?"; side "Side ?"; feedback "With feedback ?"
      mask help: Write Digital Output onto I/O channel.
      mask init:
      | NsiIo_DigitalOutput_InitializationFcn();
      settings: OpenFcn=NsiIo_DigitalOutput_OpenFcn();
      mask Help:
      | eval('block=get_param(gcb, ''RTWdata'');')
      | web([docroot '\toolbox\MUXlink\html\blocks/' block.MUXlink_BlockType '.html'])
      mask Callback channel: NsiIo_DigitalOutput_ApplyFcn(1);
      mask TypeOptions side: High | Low
      mask Callback side: NsiIo_DigitalOutput_ApplyFcn(2);
      mask Callback feedback: NsiIo_DigitalOutput_ApplyFcn(3);
      mask Display: image(imread('nsi.bmp'));text(0.5, 0.2, 'DigitalOutput_5', 'horizontalAlignment', 'center', 'verticalAlignment', 'base');plot([0.05 0.05 0.05 0.05 0.05 0.05 0.05 0.05 0.05 0.05]);port_label('input', 1, 'M3 : High Side');
  DigitalOutput8 : S-Function  FunctionName=NsiIo_DigitalOutput  Parameters=channel,side,feedback  SFunctionDeploymentMode=off  EnableBusSupport=off  mask(MUXlink I/O Digital Output){channel=2, side=High, feedback=off}
      mask prompts: channel "Channel ?"; side "Side ?"; feedback "With feedback ?"
      mask help: Write Digital Output onto I/O channel.
      mask init:
      | NsiIo_DigitalOutput_InitializationFcn();
      settings: OpenFcn=NsiIo_DigitalOutput_OpenFcn();
      mask Help:
      | eval('block=get_param(gcb, ''RTWdata'');')
      | web([docroot '\toolbox\MUXlink\html\blocks/' block.MUXlink_BlockType '.html'])
      mask Callback channel: NsiIo_DigitalOutput_ApplyFcn(1);
      mask TypeOptions side: High | Low
      mask Callback side: NsiIo_DigitalOutput_ApplyFcn(2);
      mask Callback feedback: NsiIo_DigitalOutput_ApplyFcn(3);
      mask Display: image(imread('nsi.bmp'));text(0.5, 0.2, 'DigitalOutput_2', 'horizontalAlignment', 'center', 'verticalAlignment', 'base');plot([0.05 0.05 0.05 0.05 0.05 0.05 0.05 0.05 0.05 0.05]);port_label('input', 1, 'G3 : High Side');
  Memory read : S-Function  FunctionName=NsiMem_Read  Parameters=name_var,type_var,size_var,tunable_var  SFunctionDeploymentMode=off  EnableBusSupport=off  mask(Memory read){name_var=MCU_Ignition, type_var=Boolean, size_var=1, tunable_var=on}
      mask prompts: name_var "Variable name :"; type_var "Type :"; size_var "Dim of table :"; tunable_var "Is Tunable By USB?"
      mask help: Reads current value of variable memory declared in the configurator block in calibration page.
      mask init:
      | NsiMem_Read_InitializationFcn();
      settings: OpenFcn=NsiMem_Read_OpenFcn();
      mask Help:
      | eval('block=get_param(gcb, ''RTWdata'');')
      | web([docroot '\toolbox\MUXlink\html\blocks/' block.MUXlink_BlockType '.html'])
      mask TypeOptions name_var: Gearing_Ratio | Wheel_Size | Brake1_High | Brake2_High | Throttle1_High | Throttle2_High | Brake1_Low | Brake2_Low | Throttle1_Low | Throttle2_Low | Max_Torque_Std | Max_Torque_Boost | MCU_Ignition | LV_Low_Voltage_Warning | MCUMotor_Temp_Warning | Target_Slip_Ratio | TC_P_Gain | MinTC_Torque | Max_Regen | Throttle_Active_Threshold | Brake_Active_Threshold | INV_Torque_limit | INV_Speed_Limit_Fwd | INV_Speed_limit_Rev | INV_DC_Link_Target | INV_DC_Link_Regen_Imax | INV_DC_Link_Discharge_Imax | INV_Regen_Torque_Limit | INV_Id_Debug | INV_Iq_debug
      mask Callback name_var: NsiMem_Read_ApplyFcn(1);
      mask TypeOptions type_var: Boolean | Signed Byte | Unsigned Byte | Signed Word | Unsigned Word | Signed Double Word | Unsigned Double Word | Single Float | Double Float
      mask Callback type_var: NsiMem_Read_ApplyFcn(2);
      mask Callback size_var: NsiMem_Read_ApplyFcn(3);
      mask Callback tunable_var: NsiMem_Read_ApplyFcn(4);
      mask Display: image(imread('nsi.bmp'));text(0.5, 0.35, 'MCU_Ignition', 'horizontalAlignment', 'center', 'verticalAlignment', 'base');plot([0.05 0.05 0.05 0.05 0.05 0.05 0.05 0.05 0.05 0.05]);port_label('output', 1, 'Read');
  UsbTx1 : S-Function  FunctionName=NsiUsb_Tx  Parameters=signame,resolution,offset,unite  SFunctionDeploymentMode=off  EnableBusSupport=off  mask(MUXlink Usb Tx){signame=TSS_OUTPUT, resolution=1, offset=0, unite=mV}
      mask prompts: signame "Signal name ?"; resolution "Resolution ?"; offset "Offset ?"; unite "Unit ?"
      mask help: Transmit a frame on the USB Channel.
      mask init:
      | NsiUsb_Tx_InitializationFcn();
      settings: OpenFcn=NsiUsb_Tx_OpenFcn();
      mask Help:
      | eval('block=get_param(gcb, ''RTWdata'');')
      | web([docroot '\toolbox\MUXlink\html\blocks/' block.MUXlink_BlockType '.html'])
      mask Callback signame: NsiUsb_Tx_ApplyFcn(1);
      mask Callback resolution: NsiUsb_Tx_ApplyFcn(2);
      mask Callback offset: NsiUsb_Tx_ApplyFcn(3);
      mask Callback unite: NsiUsb_Tx_ApplyFcn(4);
      mask Display: image(imread('nsi.bmp'));text(0.5, 0.2, 'USB Tx', 'horizontalAlignment', 'center', 'verticalAlignment', 'base');plot([0.05 0.05 0.05 0.05 0.05 0.05 0.05 0.05 0.05 0.05]);port_label('input',1, 'TSS_OUTPUT');
  wires:
  PostPL_Data/1 -> Bus Selector/1
  Bus Selector/5 -> DigitalOutput3/1  "<Buzzer>"
  Bus Selector/6 -> AnalogOutput1/1  "<ECU_Ok>"
  Bus Selector/7 -> AnalogOutput2/1, UsbTx1/1  "<TSS>"
  Bus Selector/4 -> DigitalOutput2/1  "<Brake_Light>"
  Bus Selector/1 -> DigitalOutput4/1, DigitalOutput6/1  "<Coolant_Enable>"
  Bus Selector/2 -> DigitalOutput7/1  "<PumpFanPower>"
  Bus Selector/3 -> DigitalOutput5/1  "<AccyFanPower>"
  Memory read/1 -> DigitalOutput8/1

== system TBRe19_ECU_Torque_request_TSS_ON/MainTask/Comms_And_Data_Output_Layer/LEDs ==
  PostPL_Data : Inport
  Bus Selector : BusSelector  OutputSignals=LEDs.RTD_LED,LEDs.X_LED,LEDs.Y_LED,LEDs.Z_LED,LEDs.APPS_LED
  DigitalOutput1 : S-Function  FunctionName=NsiIo_DigitalOutput  Parameters=channel,side,feedback  SFunctionDeploymentMode=off  EnableBusSupport=off  mask(MUXlink I/O Digital Output){channel=4, side=Low, feedback=off}
      mask prompts: channel "Channel ?"; side "Side ?"; feedback "With feedback ?"
      mask help: Write Digital Output onto I/O channel.
      mask init:
      | NsiIo_DigitalOutput_InitializationFcn();
      settings: OpenFcn=NsiIo_DigitalOutput_OpenFcn();
      mask Help:
      | eval('block=get_param(gcb, ''RTWdata'');')
      | web([docroot '\toolbox\MUXlink\html\blocks/' block.MUXlink_BlockType '.html'])
      mask Callback channel: NsiIo_DigitalOutput_ApplyFcn(1);
      mask TypeOptions side: High | Low
      mask Callback side: NsiIo_DigitalOutput_ApplyFcn(2);
      mask Callback feedback: NsiIo_DigitalOutput_ApplyFcn(3);
      mask Display: image(imread('nsi.bmp'));text(0.5, 0.2, 'DigitalOutput_4', 'horizontalAlignment', 'center', 'verticalAlignment', 'base');plot([0.05 0.05 0.05 0.05 0.05 0.05 0.05 0.05 0.05 0.05]);port_label('input', 1, 'E4 : Low Side');
  DigitalOutput2 : S-Function  FunctionName=NsiIo_DigitalOutput  Parameters=channel,side,feedback  SFunctionDeploymentMode=off  EnableBusSupport=off  mask(MUXlink I/O Digital Output){channel=3, side=Low, feedback=off}
      mask prompts: channel "Channel ?"; side "Side ?"; feedback "With feedback ?"
      mask help: Write Digital Output onto I/O channel.
      mask init:
      | NsiIo_DigitalOutput_InitializationFcn();
      settings: OpenFcn=NsiIo_DigitalOutput_OpenFcn();
      mask Help:
      | eval('block=get_param(gcb, ''RTWdata'');')
      | web([docroot '\toolbox\MUXlink\html\blocks/' block.MUXlink_BlockType '.html'])
      mask Callback channel: NsiIo_DigitalOutput_ApplyFcn(1);
      mask TypeOptions side: High | Low
      mask Callback side: NsiIo_DigitalOutput_ApplyFcn(2);
      mask Callback feedback: NsiIo_DigitalOutput_ApplyFcn(3);
      mask Display: image(imread('nsi.bmp'));text(0.5, 0.2, 'DigitalOutput_3', 'horizontalAlignment', 'center', 'verticalAlignment', 'base');plot([0.05 0.05 0.05 0.05 0.05 0.05 0.05 0.05 0.05 0.05]);port_label('input', 1, 'E3 : Low Side');
  DigitalOutput3 : S-Function  FunctionName=NsiIo_DigitalOutput  Parameters=channel,side,feedback  SFunctionDeploymentMode=off  EnableBusSupport=off  mask(MUXlink I/O Digital Output){channel=5, side=Low, feedback=off}
      mask prompts: channel "Channel ?"; side "Side ?"; feedback "With feedback ?"
      mask help: Write Digital Output onto I/O channel.
      mask init:
      | NsiIo_DigitalOutput_InitializationFcn();
      settings: OpenFcn=NsiIo_DigitalOutput_OpenFcn();
      mask Help:
      | eval('block=get_param(gcb, ''RTWdata'');')
      | web([docroot '\toolbox\MUXlink\html\blocks/' block.MUXlink_BlockType '.html'])
      mask Callback channel: NsiIo_DigitalOutput_ApplyFcn(1);
      mask TypeOptions side: High | Low
      mask Callback side: NsiIo_DigitalOutput_ApplyFcn(2);
      mask Callback feedback: NsiIo_DigitalOutput_ApplyFcn(3);
      mask Display: image(imread('nsi.bmp'));text(0.5, 0.2, 'DigitalOutput_5', 'horizontalAlignment', 'center', 'verticalAlignment', 'base');plot([0.05 0.05 0.05 0.05 0.05 0.05 0.05 0.05 0.05 0.05]);port_label('input', 1, 'K3 : Low Side');
  DigitalOutput4 : S-Function  FunctionName=NsiIo_DigitalOutput  Parameters=channel,side,feedback  SFunctionDeploymentMode=off  EnableBusSupport=off  mask(MUXlink I/O Digital Output){channel=6, side=Low, feedback=off}
      mask prompts: channel "Channel ?"; side "Side ?"; feedback "With feedback ?"
      mask help: Write Digital Output onto I/O channel.
      mask init:
      | NsiIo_DigitalOutput_InitializationFcn();
      settings: OpenFcn=NsiIo_DigitalOutput_OpenFcn();
      mask Help:
      | eval('block=get_param(gcb, ''RTWdata'');')
      | web([docroot '\toolbox\MUXlink\html\blocks/' block.MUXlink_BlockType '.html'])
      mask Callback channel: NsiIo_DigitalOutput_ApplyFcn(1);
      mask TypeOptions side: High | Low
      mask Callback side: NsiIo_DigitalOutput_ApplyFcn(2);
      mask Callback feedback: NsiIo_DigitalOutput_ApplyFcn(3);
      mask Display: image(imread('nsi.bmp'));text(0.5, 0.2, 'DigitalOutput_6', 'horizontalAlignment', 'center', 'verticalAlignment', 'base');plot([0.05 0.05 0.05 0.05 0.05 0.05 0.05 0.05 0.05 0.05]);port_label('input', 1, 'K4 : Low Side');
  DigitalOutput5 : S-Function  FunctionName=NsiIo_DigitalOutput  Parameters=channel,side,feedback  SFunctionDeploymentMode=off  EnableBusSupport=off  mask(MUXlink I/O Digital Output){channel=2, side=Low, feedback=off}
      mask prompts: channel "Channel ?"; side "Side ?"; feedback "With feedback ?"
      mask help: Write Digital Output onto I/O channel.
      mask init:
      | NsiIo_DigitalOutput_InitializationFcn();
      settings: OpenFcn=NsiIo_DigitalOutput_OpenFcn();
      mask Help:
      | eval('block=get_param(gcb, ''RTWdata'');')
      | web([docroot '\toolbox\MUXlink\html\blocks/' block.MUXlink_BlockType '.html'])
      mask Callback channel: NsiIo_DigitalOutput_ApplyFcn(1);
      mask TypeOptions side: High | Low
      mask Callback side: NsiIo_DigitalOutput_ApplyFcn(2);
      mask Callback feedback: NsiIo_DigitalOutput_ApplyFcn(3);
      mask Display: image(imread('nsi.bmp'));text(0.5, 0.2, 'DigitalOutput_2', 'horizontalAlignment', 'center', 'verticalAlignment', 'base');plot([0.05 0.05 0.05 0.05 0.05 0.05 0.05 0.05 0.05 0.05]);port_label('input', 1, 'H3 : Low Side');
  wires:
  Bus Selector/2 -> DigitalOutput1/1  "<X_LED>"
  PostPL_Data/1 -> Bus Selector/1
  Bus Selector/1 -> DigitalOutput2/1  "<RTD_LED>"
  Bus Selector/3 -> DigitalOutput3/1  "<Y_LED>"
  Bus Selector/4 -> DigitalOutput4/1  "<Z_LED>"
  Bus Selector/5 -> DigitalOutput5/1  "<APPS_LED>"
